simulink model "chap3_3sim"  (Simulink 7.7)
settings: Solver=ode5  StartTime=0.0  StopTime=10  FixedStep=0.001  RelTol=1e-3
settings Model: Creator=ljk  LastModifiedBy=ljk  ExtModeTrigMode=oneshot  ExtModeArmWhenConnect=off
settings DataIOCC: LimitDataPoints=off  SignalLoggingName=sigsOut
settings OptimizationCC: BooleanDataType=off
settings DebuggingCC: SaveWithParameterizedLinksMsg=none  SignalResolutionControl=TryResolveAllWithWarning  SolverPrmCheckMsg=none  MultiTaskDSMMsg=warning  MultiTaskCondExecSysMsg=none  StrictBusMsg=None
settings HardwareCC: TargetUnknown=on
settings RTWCC: IncludeERTFirstTime=on

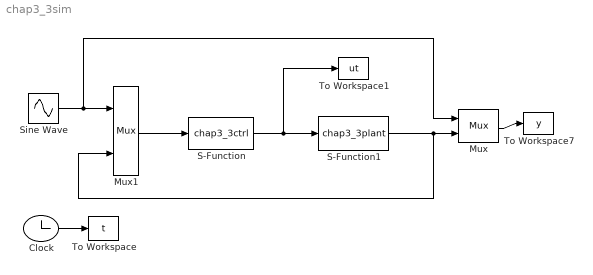
== system chap3_3sim ==
  Clock : Clock
  Mux : Mux  Inputs=2
  Mux1 : Mux  Inputs=2
  S-Function : S-Function  FunctionName=chap3_3ctrl  EnableBusSupport=off
  S-Function1 : S-Function  FunctionName=chap3_3plant  EnableBusSupport=off
  Sine Wave : Sin  SampleTime=0
  To Workspace : ToWorkspace  VariableName=t  SampleTime=-1  SaveFormat=Array
  To Workspace1 : ToWorkspace  VariableName=ut  SampleTime=-1  SaveFormat=Array
  To Workspace7 : ToWorkspace  VariableName=y  SampleTime=-1  SaveFormat=Array
  wires:
  Mux1/1 -> S-Function/1
  S-Function/1 -> S-Function1/1, To Workspace1/1
  S-Function1/1 -> Mux1/2, Mux/2
  Mux/1 -> To Workspace7/1
  Sine Wave/1 -> Mux/1, Mux1/1
  Clock/1 -> To Workspace/1
